simulink model "smd_model"  (R2015a)
settings: Solver=ode15s  StartTime=0.0  StopTime=200  RelTol=1e-3
settings Model: Creator=Arnab Banerjee  LastModifiedBy=Arnab Banerjee

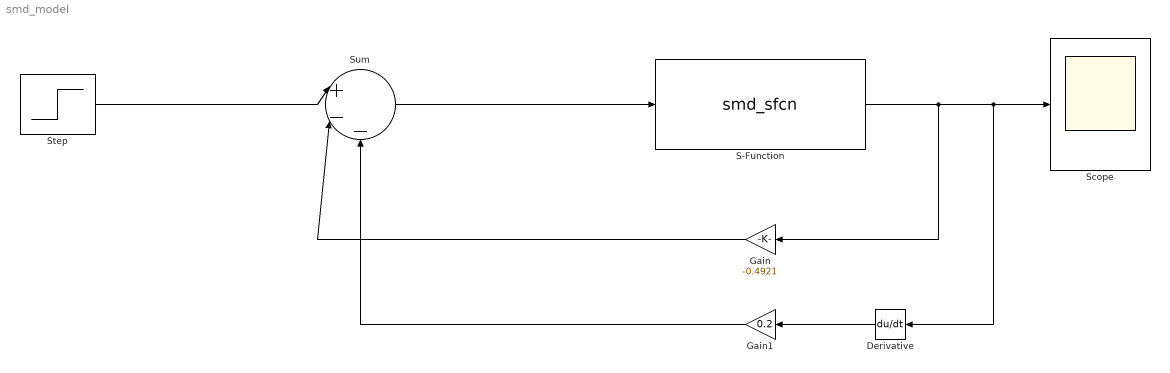
== system smd_model ==
  Derivative : Derivative
  Gain : Gain  Gain=-0.4921
  Gain1 : Gain  Gain=0.2
  S-Function : S-Function  FunctionName=smd_sfcn
  Scope : Scope
      settings: TimeRange=40
  Step : Step  Time=0  After=0.5  SampleTime=0
  Sum : Sum  Inputs=|+--
  wires:
  S-Function/1 -> Gain/1, Derivative/1, Scope/1
  Step/1 -> Sum/1
  Sum/1 -> S-Function/1
  Gain/1 -> Sum/2
  Derivative/1 -> Gain1/1
  Gain1/1 -> Sum/3
